simulink subsystem "PvtSubSys_VSM_TLS"  (R2020b)
settings: Solver=VariableStepAuto  StartTime=0.0  StopTime=10.0  RelTol=1e-3
undefined symbols (not defined in the file or in its folder): HWA_STATE, LCK_STATE, P_VSM_TLS_LCCancelTime
libraries: simulink x18
settings Model: Creator=GW00133806  LastModifiedBy=GW00201118

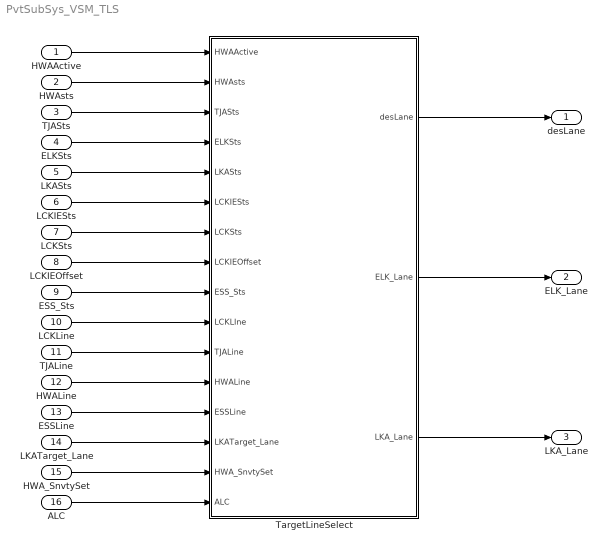
== system PvtSubSys_VSM_TLS ==
  HWAActive : Inport  Description=b|HWA激活状态
  HWAsts : Inport  Description=|  Port=2  OutDataTypeStr=Enum: HWA_STATE
      | uint8|HWA状态：0-OFF;1-Idle;2-Ready;3-CCAct（巡航）;4-Pause;5-LeftTurn;6-RightTurn;
      | 7-Error;9-SafeStop;10-SlowRetreat
  TJASts : Inport  Description=|  Port=3  OutDataTypeStr=Enum: TJA_STATE
      | uint8|TJS状态：0-Off;1-Idle;2-Ready;3-Active;6-wait;7-Error;9-SafeStop;
      | 10-SlowRetreat.
  "ELKSts " : Inport  Description=|  Port=4  OutDataTypeStr=Enum: ELKSTATE
      | uint8|ELK状态：0-ELK_OFF;1-ELK_IDLE;2-ELK_READY;3_ELK_ACTIVE_LEFT;4-ELK_ACTIVE_RIGHT;
      | 5-ELK_OnComing_LEFT;6-ELK_OnComing_RIGHT;7-ELK_OVERTAKING_LEFT;
      | 8-ELK_OVERTAKING_RIGHT;9-ELK_ERROR;10-ELK_DEFAULT;
  LKASts : Inport  Description=|  Port=5  OutDataTypeStr=Enum: STATE
      | uint8|LKA状态：0-OFF;1-IDLE;2-READY;3-ACTIVE;4-ACTIVE_LEFT;5-ACTIVE_RIGHT;
      | 6-ERROR;7-DEFAULT.
  LCKIESts : Inport  Description=|  Port=6  OutDataTypeStr=Enum: STATE
      | uint8|LCKIE状态：0-OFF;1-IDLE;2-READY;3-ACTIVE;4-ACTIVE_LEFT;5-ACTIVE_RIGHT;
      | 6-ERROR;7-DEFAULT.
  LCKSts : Inport  Description=uint8|LCK状态：0-LCK_OFF;1-LCK_Idle;2-LCK_Ready;3-LCK_Active;7-LCK_Errror.  Port=7  OutDataTypeStr=Enum: LCK_STATE
  LCKIEOffset : Inport  Description=m|LCKIE车道线C0偏移量  Port=8
  "ESS_Sts " : Inport  Description=|  Port=9
      | uint8|ESS状态：0-Off;1-IDLE;2-Ready;3-Active;4-Active_LEFT;5-Active_Right;
      | 6-Error.
  LCKLine : Inport  Port=10  OutDataTypeStr=Bus: LSM_LCK_BUS
  TJALine : Inport  Port=11  OutDataTypeStr=Bus: LSM_TJA_ICA_BUS
  HWALine : Inport  Port=12  OutDataTypeStr=Bus: LSM_HWA_BUS
  ESSLine : Inport  Port=13  OutDataTypeStr=Bus: LSM_ESS_BUS
  "LKATarget_Lane " : Inport  Port=14  OutDataTypeStr=Bus: LaneARe_SP
  HWA_SnvtySet : Inport  Description=uint8|HWA换道灵敏度  Port=15
  ALC : Inport  Description=|  Port=16
      | bus|PLAN发的总线信号："HMI提示信息驱动信号；0x1 换道完成请关闭转向灯
      | 0x2 换道取消;0x3 换道超时;0x4 换道速度过低;0x5 即将向左超车;0x6 即将向右超车
      | 0x7 车速过高不可换道"
  TargetLineSelect : Subsystem
  desLane : Outport  Description=|目标车道线信息  OutDataTypeStr=Bus: TLS_DesLane
  ELK_Lane : Outport  Description=|ELK车道线信息  Port=2  OutDataTypeStr=Bus: TLS_ELKLane
  LKA_Lane : Outport  Description=|LKA车道线信息  Port=3  OutDataTypeStr=Bus: TLS_LKALane
  wires:
  HWAActive/1 -> TargetLineSelect/1(HWAActive)
  HWAsts/1 -> TargetLineSelect/2(HWAsts)
  TargetLineSelect/3(LKA_Lane) -> LKA_Lane/1
  "ESS_Sts "/1 -> TargetLineSelect/9("ESS_Sts ")
  "LKATarget_Lane "/1 -> TargetLineSelect/14("LKATarget_Lane ")
  TJASts/1 -> TargetLineSelect/3(TJASts)
  LKASts/1 -> TargetLineSelect/5(LKASts)
  LCKLine/1 -> TargetLineSelect/10(LCKLIne)
  LCKSts/1 -> TargetLineSelect/7(LCKSts)
  LCKIESts/1 -> TargetLineSelect/6(LCKIESts)
  LCKIEOffset/1 -> TargetLineSelect/8(LCKIEOffset)
  TJALine/1 -> TargetLineSelect/11(TJALine)
  TargetLineSelect/2(ELK_Lane) -> ELK_Lane/1
  "ELKSts "/1 -> TargetLineSelect/4("ELKSts ")
  TargetLineSelect/1(desLane) -> desLane/1
  ESSLine/1 -> TargetLineSelect/13(ESSLine)
  HWALine/1 -> TargetLineSelect/12(HWALine)
  HWA_SnvtySet/1 -> TargetLineSelect/15(HWA_SnvtySet)
  ALC/1 -> TargetLineSelect/16(ALC)

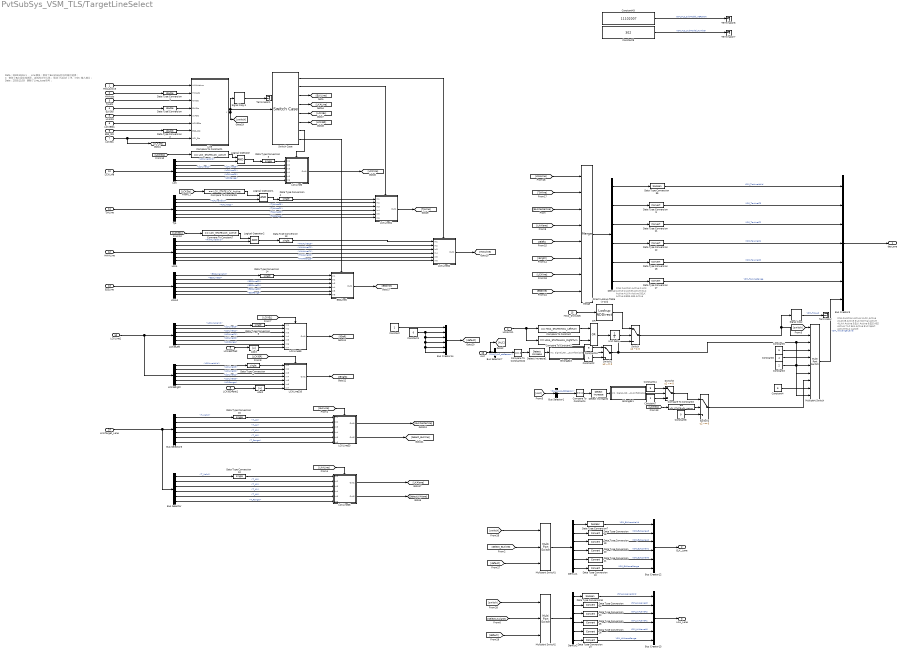
== system PvtSubSys_VSM_TLS/TargetLineSelect ==
  note: 0:No Function Active
      | 1:LCK Active
      | 2:LCKIE Active
      | 3:LC Normal Active
      | 4:LKA Active
      | 5:ELK Active
      | 6:ESS AES Active
      | 7:LC Eco Active
      | 8:LC Sport Active
      | 9:LC cancel
  note: Data：2020/10/15
      | 1、Line模块：修改了ELKstate对应的输出选择；
      | 2、修改了ELK目标线选择，边线改为中心线；
      | 取消了fusion（re、line）输入接口；
      | Data：2020/11/03
      | 删除了Line_type信号；
  note: 0:No Function Active
      | 1:LCK Active
      | 2:LCKIE Active
      | 3:LC Active
      | 4:LKA Active
      | 5:ELK Active
      | 6:ESS AES Active
  HWAActive : Inport  OutDataTypeStr=boolean
  HWAsts : Inport  Port=2
  TJASts : Inport  Port=3
  "ELKSts " : Inport  Port=4
  LKASts : Inport  Port=5
  LCKIESts : Inport  Port=6
  LCKSts : Inport  Port=7
  LCKIEOffset : Inport  Port=8  OutDataTypeStr=single
  "ESS_Sts " : Inport  Port=9  OutDataTypeStr=uint8
  LCKLIne : Inport  Port=10
  TJALine : Inport  Port=11
  HWALine : Inport  Port=12
  ESSLine : Inport  Port=13
  "LKATarget_Lane " : Inport  Port=14
  HWA_SnvtySet : Inport  Port=15
  ALC : Inport  Port=16
  Abs2 : Abs
  Abs3 : Abs
  Bus Creator12 : BusCreator  Inputs=6
  Bus Creator13 : BusCreator  Inputs=6
  Bus Creator14 : BusCreator  Inputs=6
  Bus Selector : BusSelector  OutputSignals=T_Valid,T_A3,T_A2,T_A1,T_A0,T_Range
  Bus Selector1 : BusSelector  OutputSignals=PLAN_ALC_stsReason
  Bus Selector3 : BusSelector  OutputSignals=T_Valid,T_A3,T_A2,T_A1,T_A0,T_Range
  Bus Selector7 : BusSelector  OutputSignals=PLAN_ALC_stsReason
  Bus Creator3 : BusCreator  Inputs=7
  Compare To Constant : simulink/Logic and Bit Operations/Compare To Constant  relop===  const=HWA_STATE.HWA_LeftTurn  OutDataTypeStr=boolean
  Compare To Constant{1,3,6..7} (4 alike) : simulink/Logic and Bit Operations/Compare To Constant  relop===  const=LCK_STATE.LCK_Active  OutDataTypeStr=boolean
  Compare To Constant102 : simulink/Logic and Bit Operations/Compare To Constant  relop===  const=2  OutDataTypeStr=boolean
  Compare To Constant2 : simulink/Logic and Bit Operations/Compare To Constant  relop===  const=HWA_STATE.HWA_RightTurn  OutDataTypeStr=boolean
  Compare To Constant4 : simulink/Logic and Bit Operations/Compare To Constant  relop===  const=2  OutDataTypeStr=boolean
  Constant : Constant  OutDataTypeStr=single
  Constant1 : Constant  Value=0  OutDataTypeStr=single
  Constant10 : Constant  Value=9  OutDataTypeStr=uint8
  Constant11 : Constant  Value=9  OutDataTypeStr=uint8
  Constant2 : Constant  OutDataTypeStr=uint8
  Constant3 : Constant  Value=2  OutDataTypeStr=uint8
  Constant4 : Constant  Value=6  OutDataTypeStr=uint8
  Constant43 : Constant  Value=11102007  OutDataTypeStr=uint32
  Constant5 : Constant  Value=5  OutDataTypeStr=uint8
  Constant6 : Constant  Value=4  OutDataTypeStr=uint8
  Constant7 : Constant  OutDataTypeStr=uint8
  Constant8 : Constant  Value=0  OutDataTypeStr=uint8
  Constant9 : Constant  Value=302  OutDataTypeStr=uint16
  Data Type Conversion : DataTypeConversion  OutDataTypeStr=double
  Data Type Conversion1 : DataTypeConversion  OutDataTypeStr=double
  Data Type Conversion{3..6,10,13..15} (8 alike) : DataTypeConversion  OutDataTypeStr=single
  Data Type Conversion{9,11..12,16..27} (15 alike) : DataTypeConversion
  Data Type Conversion2 : DataTypeConversion  OutDataTypeStr=double
  Data Type Conversion35 : DataTypeConversion  OutDataTypeStr=boolean
  Data Type Conversion7 : DataTypeConversion  OutDataTypeStr=boolean
  Data Type Conversion8 : DataTypeConversion  OutDataTypeStr=boolean
  Demux : Demux  Outputs=6
  Demux1 : Demux  Outputs=6
  Demux2 : Demux  Outputs=6
  Detect Increase1 : simulink/Logic and Bit Operations/Detect Increase  vinit=0.0  OutDataTypeStr=boolean
  Detect Increase2 : simulink/Logic and Bit Operations/Detect Increase  vinit=0.0  OutDataTypeStr=boolean
  Direct Lookup Table (n-D)2 : LookupNDDirect  NumberOfTableDimensions=1  Table=[3 8 7]  TableDataTypeStr=uint8
  ESSLineS : Subsystem  TreatAsAtomicUnit=on
  Enlong3s1 : Subsystem
  Enlong3s3 : Subsystem
  HWA : BusSelector  OutputSignals=HWALineValid,HWALineC3,HWALineC2,HWALineC1,HWALineC0,HWARange
  HWA2 : BusSelector  OutputSignals=ESSLineValid,ESSLineC3,ESSLineC2,ESSLineC1,ESSLineC0,ESSRange
  HWAsts1 : InportShadow  Port=2
  LCK : BusSelector  OutputSignals=LCKLineValid,LCKLineC3,LCKLineC2,LCKLineC1,LCKLineC0,LCKRange
  LCKIELeft : BusSelector  OutputSignals=LCKLineValid,LCKLineC3,LCKLineC2,LCKLineC1,LCKLineC0,LCKRange
  LCKIEOffset1 : InportShadow  Port=8  OutDataTypeStr=single
  LCKIERight : BusSelector  OutputSignals=LCKLineValid,LCKLineC3,LCKLineC2,LCKLineC1,LCKLineC0,LCKRange
  LCKLIne1 : InportShadow  Port=10
  LCKLineS : Subsystem  TreatAsAtomicUnit=on
  LCKLineS1 : Subsystem  TreatAsAtomicUnit=on
  LCKLineS10 : Subsystem  TreatAsAtomicUnit=on
  LCKLineS2 : Subsystem  TreatAsAtomicUnit=on
  LCKLineS3 : Subsystem  TreatAsAtomicUnit=on
  LCKLineS6 : Subsystem  TreatAsAtomicUnit=on
  LCKLineS9 : Subsystem  TreatAsAtomicUnit=on
  Line : MATLAB Function  TreatAsAtomicUnit=on
  Logical Operator : Logic  AllPortsSameDT=off  OutDataTypeStr=boolean
  Logical Operator1 : Logic  AllPortsSameDT=off  OutDataTypeStr=boolean
  Logical Operator2 : Logic  AllPortsSameDT=off  OutDataTypeStr=boolean
  Merge : Merge  Inputs=8
  Multiport Switch : MultiPortSwitch  Inputs=9
  Multiport Switch1 : MultiPortSwitch  DataPortOrder=Specify indices  Inputs=4  DataPortIndices={3,7}  DiagnosticForDefault=None
  Multiport Switch2 : MultiPortSwitch  DataPortOrder=Specify indices  Inputs=4  DataPortIndices={7,8}  DiagnosticForDefault=None
  OR : Logic  Operator=OR  AllPortsSameDT=off  OutDataTypeStr=boolean
  Signal Copy : SignalConversion  OverrideOpt=off
  Signal Copy1 : SignalConversion  OverrideOpt=off
  Switch{,1..3} (4 alike) : Switch  Criteria=u2 ~= 0
  Switch Case : SwitchCase  CaseConditions={1,2,3,4,5,6,7,8}  ShowDefaultCase=off
  TJA : BusSelector  OutputSignals=TJALineValid,TJALineC3,TJALineC2,TJALineC1,TJALineC0,TJARange
  Terminator{,1,6..7} (4 alike) : Terminator
  Unit Delay : UnitDelay  SampleTime=-1  HasFrameUpgradeWarning=on
  desLane : Outport
  ELK_Lane : Outport  Port=2
  LKA_Lane : Outport  Port=3
  wires:
  Constant2/1 -> Switch2/3
  Detect Increase1/1 -> Enlong3s3/1(In1)
  Constant10/1 -> Switch2/1
  Enlong3s3/1(Signal_NOH_SysInfoDisplay) -> Switch2/2
  Bus Selector7/1 -> Compare To Constant102/1  "<PLAN_ALC_stsReason>"
  ALC/1 -> Bus Selector7/1, [ALC]
  Compare To Constant102/1 -> Detect Increase1/1
  Switch3/1 -> Switch1/1
  Constant7/1 -> Switch3/3
  Detect Increase2/1 -> Enlong3s1/1(In1)
  Constant11/1 -> Switch3/1
  Enlong3s1/1(Signal_NOH_SysInfoDisplay) -> Switch3/2
  Bus Selector1/1 -> Compare To Constant4/1  "<PLAN_ALC_stsReason>"
  [ALC] -> Bus Selector1/1
  Compare To Constant4/1 -> Detect Increase2/1
  Signal Copy1/1 -> Terminator1/1
  Signal Copy/1 -> Terminator/1  "VSM_TLS_LC"
  Switch/1 -> Multiport Switch/2, Signal Copy/1
  Constant43/1 -> Terminator6/1  "VSM_TLS_SubModel_VERSION"
  Constant9/1 -> Terminator7/1  "VSM_TLS_SubModel_Number"
  HWA_SnvtySet/1 -> Direct Lookup Table (n-D)2/1
  Data Type Conversion8/1 -> Bus Creator13/1  "VSM_LKALaneValid"
  Data Type Conversion7/1 -> Bus Creator12/1  "VSM_ELKLaneValid"
  Data Type Conversion2/1 -> Line/7(ESS_Sts)
  LCKLIne1/1 -> LCKIELeft/1, LCKIERight/1
  ESSLine/1 -> HWA2/1
  HWALine/1 -> HWA/1
  TJALine/1 -> TJA/1
  [SelectLKAlane] -> Multiport Switch2/2
  LCKLineS6/2(Out2) -> [SelectLKAlane]
  Demux/1 -> Data Type Conversion35/1
  Switch Case/7 -> LCKLineS/Action
  Data Type Conversion10/1 -> LCKLineS6/1(In1)
  Bus Selector/6 -> LCKLineS6/6(In6)  "<T_Range>"
  Bus Selector/5 -> LCKLineS6/5(In5)  "<T_A0>"
  Bus Selector/4 -> LCKLineS6/4(In4)  "<T_A1>"
  Bus Selector/3 -> LCKLineS6/3(In3)  "<T_A2>"
  Bus Selector/2 -> LCKLineS6/2(In2)  "<T_A3>"
  Bus Selector/1 -> Data Type Conversion10/1  "<T_Valid>"
  ESSLineS/1(Out1) -> [ESSline]
  Data Type Conversion14/1 -> ESSLineS/1(In1)
  Switch Case/8 -> ESSLineS/Action
  HWA2/6 -> ESSLineS/6(In6)  "<ESSRange>"
  HWA2/5 -> ESSLineS/5(In5)  "<ESSLineC0>"
  HWA2/4 -> ESSLineS/4(In4)  "<ESSLineC1>"
  HWA2/3 -> ESSLineS/3(In3)  "<ESSLineC2>"
  HWA2/2 -> ESSLineS/2(In2)  "<ESSLineC3>"
  HWA2/1 -> Data Type Conversion14/1  "<ESSLineValid>"
  "ESS_Sts "/1 -> Data Type Conversion2/1
  LCKLineS3/2(Out2) -> [Select_ELKline]
  [ELKCenterline] -> Merge/3
  [TJAline] -> Merge/2
  [HWAline] -> Merge/1
  Merge/1 -> Demux/1
  LCKLineS6/1(Out1) -> [LKAlane]
  LCKLineS3/1(Out1) -> [ELKCenterline]
  LCKLineS10/1(Out1) -> [IEright]
  LCKLineS9/1(Out1) -> [IEleft]
  LCKLineS2/1(Out1) -> [HWAline]
  LCKLineS1/1(Out1) -> [TJAline]
  LCKLineS/1(Out1) -> [LCKline]
  [default] -> Multiport Switch2/3
  [switch] -> Multiport Switch2/1
  [default] -> Multiport Switch1/3
  Bus Creator14/1 -> [default]
  Constant1/1 -> Bus Creator14/2, Bus Creator14/4, Bus Creator14/6, Bus Creator14/5, Bus Creator14/3
  Constant/1 -> Bus Creator14/1
  [switch] -> Multiport Switch1/1
  Line/1(y) -> [switch], Switch Case/1, Signal Copy1/1
  Data Type Conversion3/1 -> LCKLineS/1(In1)
  Logical Operator/1 -> Data Type Conversion3/1
  Bus Creator12/1 -> ELK_Lane/1
  LCK/1 -> Logical Operator/2  "<LCKLineValid>"
  Bus Creator13/1 -> LKA_Lane/1
  Demux2/6 -> Data Type Conversion27/1
  Demux2/5 -> Data Type Conversion26/1
  Demux2/4 -> Data Type Conversion25/1
  Demux2/3 -> Data Type Conversion24/1
  Demux2/2 -> Data Type Conversion23/1
  Demux2/1 -> Data Type Conversion8/1
  Multiport Switch2/1 -> Demux2/1
  Demux1/6 -> Data Type Conversion22/1
  Demux1/5 -> Data Type Conversion21/1
  Demux1/4 -> Data Type Conversion20/1
  Demux1/3 -> Data Type Conversion19/1
  Demux1/2 -> Data Type Conversion18/1
  Demux1/1 -> Data Type Conversion7/1
  Multiport Switch1/1 -> Demux1/1
  [Select_ELKline] -> Multiport Switch1/2
  Abs3/1 -> LCKLineS9/7(In7)
  Abs2/1 -> LCKLineS10/7(In7)
  Data Type Conversion1/1 -> Line/2(HWAsts)
  HWAsts/1 -> Data Type Conversion1/1
  LCKIEOffset/1 -> Abs3/1
  Data Type Conversion35/1 -> Bus Creator3/1  "VSM_TarLineValid"
  Data Type Conversion13/1 -> LCKLineS2/1(In1)
  Data Type Conversion6/1 -> LCKLineS10/1(In1)
  Data Type Conversion5/1 -> LCKLineS9/1(In1)
  Data Type Conversion4/1 -> LCKLineS1/1(In1)
  Compare To Constant1/1 -> Logical Operator/1
  [LCKIER] -> LCKLineS10/Action
  [LCKIEL] -> LCKLineS9/Action
  [LKALine] -> LCKLineS6/Action
  [ELKLine] -> LCKLineS3/Action
  Switch Case/3 -> [ELKLine]
  Data Type Conversion/1 -> Line/4(ELKSts)
  LCKIESts/1 -> Line/6(LCKIESts)
  LKASts/1 -> Line/5(LKASts)
  "ELKSts "/1 -> Data Type Conversion/1
  LCKIEOffset1/1 -> Abs2/1
  LCKIERight/6 -> LCKLineS10/6(In6)  "<LCKRange>"
  LCKIERight/4 -> LCKLineS10/4(In4)  "<LCKLineC1>"
  LCKIERight/3 -> LCKLineS10/3(In3)  "<LCKLineC2>"
  LCKIERight/1 -> Data Type Conversion6/1  "<LCKLineValid>"
  LCKIERight/5 -> LCKLineS10/5(In5)  "<LCKLineC0>"
  LCKIERight/2 -> LCKLineS10/2(In2)  "<LCKLineC3>"
  LCKIELeft/6 -> LCKLineS9/6(In6)  "<LCKRange>"
  LCKIELeft/1 -> Data Type Conversion5/1  "<LCKLineValid>"
  LCKIELeft/3 -> LCKLineS9/3(In3)  "<LCKLineC2>"
  LCKIELeft/5 -> LCKLineS9/5(In5)  "<LCKLineC0>"
  LCKIELeft/2 -> LCKLineS9/2(In2)  "<LCKLineC3>"
  LCKIELeft/4 -> LCKLineS9/4(In4)  "<LCKLineC1>"
  LCKLIne/1 -> LCK/1
  LCK/6 -> LCKLineS/6(In6)  "<LCKRange>"
  LCK/2 -> LCKLineS/2(In2)  "<LCKLineC3>"
  LCK/4 -> LCKLineS/4(In4)  "<LCKLineC1>"
  LCK/5 -> LCKLineS/5(In5)  "<LCKLineC0>"
  LCK/3 -> LCKLineS/3(In3)  "<LCKLineC2>"
  TJA/5 -> LCKLineS1/5(In5)  "<TJALineC0>"
  TJA/4 -> LCKLineS1/4(In4)  "<TJALineC1>"
  TJA/2 -> LCKLineS1/2(In2)  "<TJALineC3>"
  TJA/1 -> Logical Operator1/2  "<TJALineValid>"
  TJA/6 -> LCKLineS1/6(In6)  "<TJARange>"
  TJA/3 -> LCKLineS1/3(In3)  "<TJALineC2>"
  HWA/1 -> Logical Operator2/2  "<HWALineValid>"
  HWA/5 -> LCKLineS2/5(In5)  "<HWALineC0>"
  HWA/3 -> LCKLineS2/3(In3)  "<HWALineC2>"
  HWA/2 -> LCKLineS2/2(In2)  "<HWALineC3>"
  HWA/6 -> LCKLineS2/6(In6)  "<HWARange>"
  Demux/3 -> Data Type Conversion11/1
  HWA/4 -> LCKLineS2/4(In4)  "<HWALineC1>"
  Demux/2 -> Data Type Conversion9/1
  Switch Case/1 -> LCKLineS2/Action
  Switch Case/2 -> LCKLineS1/Action
  Demux/4 -> Data Type Conversion12/1
  Bus Creator3/1 -> desLane/1
  HWAActive/1 -> Line/1(HWAActive)
  TJASts/1 -> Line/3(TJASts)
  Demux/5 -> Data Type Conversion16/1
  Demux/6 -> Data Type Conversion17/1
  Compare To Constant6/1 -> Logical Operator1/1
  Logical Operator1/1 -> Data Type Conversion4/1
  Compare To Constant7/1 -> Logical Operator2/1
  Logical Operator2/1 -> Data Type Conversion13/1
  "LKATarget_Lane "/1 -> Bus Selector3/1, Bus Selector/1
  Bus Selector3/1 -> Data Type Conversion15/1  "<T_Valid>"
  Bus Selector3/2 -> LCKLineS3/2(In2)  "<T_A3>"
  Bus Selector3/3 -> LCKLineS3/3(In3)  "<T_A2>"
  Bus Selector3/4 -> LCKLineS3/4(In4)  "<T_A1>"
  Bus Selector3/5 -> LCKLineS3/5(In5)  "<T_A0>"
  Bus Selector3/6 -> LCKLineS3/6(In6)  "<T_Range>"
  Switch Case/4 -> [LKALine]
  Switch Case/5 -> [LCKIEL]
  Switch Case/6 -> [LCKIER]
  [LKAlane] -> Merge/4
  [IEleft] -> Merge/5
  [IEright] -> Merge/6
  [LCKline] -> Merge/7
  [ESSline] -> Merge/8
  Data Type Conversion15/1 -> LCKLineS3/1(In1)
  Multiport Switch/1 -> Bus Creator3/7  "VSM_TarDangerLevel"
  Switch2/1 -> Multiport Switch/3, Multiport Switch/10, Switch/3
  Constant3/1 -> Multiport Switch/7, Multiport Switch/6
  Constant4/1 -> Multiport Switch/9
  Constant5/1 -> Multiport Switch/4
  Constant6/1 -> Multiport Switch/5
  LCKSts/1 -> [LCKSts], Line/8(LCK_Sts)
  [LCKSts] -> Compare To Constant1/1
  [LCKSts] -> Compare To Constant6/1
  [LCKSts] -> Compare To Constant7/1
  Data Type Conversion9/1 -> Bus Creator3/2  "VSM_TarLineC3"
  Data Type Conversion11/1 -> Bus Creator3/3  "VSM_TarLineC2"
  Data Type Conversion12/1 -> Bus Creator3/4  "VSM_TarLineC1"
  Data Type Conversion16/1 -> Bus Creator3/5  "VSM_TarLineC0"
  Data Type Conversion17/1 -> Bus Creator3/6  "VSM_TarLineRange"
  Data Type Conversion18/1 -> Bus Creator12/2  "VSM_ELKLaneA3"
  Data Type Conversion19/1 -> Bus Creator12/3  "VSM_ELKLaneA2"
  Data Type Conversion20/1 -> Bus Creator12/4  "VSM_ELKLaneA1"
  Data Type Conversion21/1 -> Bus Creator12/5  "VSM_ELKLaneA0"
  Data Type Conversion22/1 -> Bus Creator12/6  "VSM_ELKLaneRange"
  Data Type Conversion23/1 -> Bus Creator13/2  "VSM_LKALaneA3"
  Data Type Conversion24/1 -> Bus Creator13/3  "VSM_LKALaneA2"
  Data Type Conversion25/1 -> Bus Creator13/4  "VSM_LKALaneA1"
  Data Type Conversion26/1 -> Bus Creator13/5  "VSM_LKALaneA0"
  Data Type Conversion27/1 -> Bus Creator13/6  "VSM_LKALaneRange"
  [switch] -> Multiport Switch/1
  HWAsts1/1 -> Compare To Constant2/1, Compare To Constant/1
  Compare To Constant/1 -> OR/1
  Compare To Constant2/1 -> OR/2
  OR/1 -> Unit Delay/1
  Direct Lookup Table (n-D)2/1 -> Switch/1
  [LCKSts] -> Compare To Constant3/1
  Compare To Constant3/1 -> Switch1/2
  Switch1/1 -> Multiport Switch/8
  Constant8/1 -> Switch1/3
  Unit Delay/1 -> Switch/2

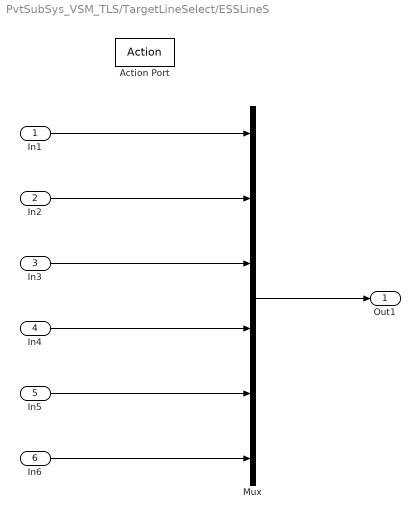
== system PvtSubSys_VSM_TLS/TargetLineSelect/ESSLineS ==
  In1 : Inport
  In2 : Inport  Port=2
  In3 : Inport  Port=3
  In4 : Inport  Port=4
  In5 : Inport  Port=5
  In6 : Inport  Port=6
  Action Port : ActionPort
  Mux : Mux  Inputs=6
  Out1 : Outport
  wires:
  In5/1 -> Mux/5
  In4/1 -> Mux/4
  In6/1 -> Mux/6
  In3/1 -> Mux/3
  In2/1 -> Mux/2
  In1/1 -> Mux/1
  Mux/1 -> Out1/1

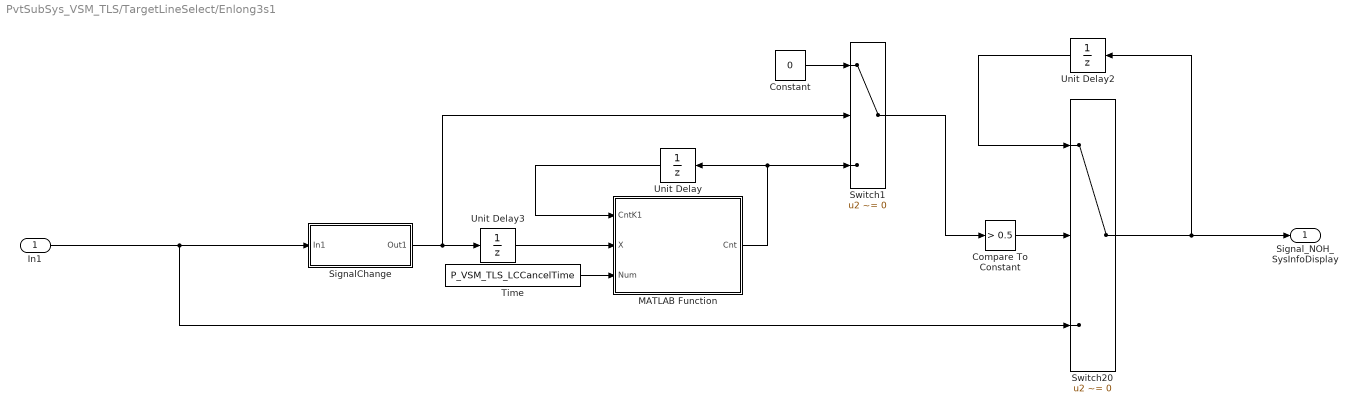
== system PvtSubSys_VSM_TLS/TargetLineSelect/Enlong3s1 ==
  In1 : Inport
  Compare To Constant : simulink/Logic and Bit Operations/Compare To Constant  relop=>  const=0.5  OutDataTypeStr=boolean
  Constant : Constant  Value=0  OutDataTypeStr=uint16
  MATLAB Function : MATLAB Function  TreatAsAtomicUnit=on
  SignalChange : Subsystem
  Switch1 : Switch  Criteria=u2 ~= 0
  Switch20 : Switch  Criteria=u2 ~= 0
  Time : Constant  Description=250  Value=P_VSM_TLS_LCCancelTime  OutDataTypeStr=uint16
      settings: AttributesFormatString=%<Description>
  Unit Delay : UnitDelay  SampleTime=-1  HasFrameUpgradeWarning=on
  Unit Delay2 : UnitDelay  SampleTime=-1  HasFrameUpgradeWarning=on
  Unit Delay3 : UnitDelay  SampleTime=-1  HasFrameUpgradeWarning=on
  Signal_NOH_SysInfoDisplay : Outport
  wires:
  In1/1 -> Switch20/3, SignalChange/1(In1)
  SignalChange/1(Out1) -> Switch1/2, Unit Delay3/1
  Unit Delay/1 -> MATLAB Function/1(CntK1)
  Constant/1 -> Switch1/1
  MATLAB Function/1(Cnt) -> Switch1/3, Unit Delay/1
  Switch1/1 -> Compare To Constant/1
  Compare To Constant/1 -> Switch20/2
  Unit Delay3/1 -> MATLAB Function/2(X)
  Unit Delay2/1 -> Switch20/1
  Switch20/1 -> Unit Delay2/1, Signal_NOH_SysInfoDisplay/1
  Time/1 -> MATLAB Function/3(Num)

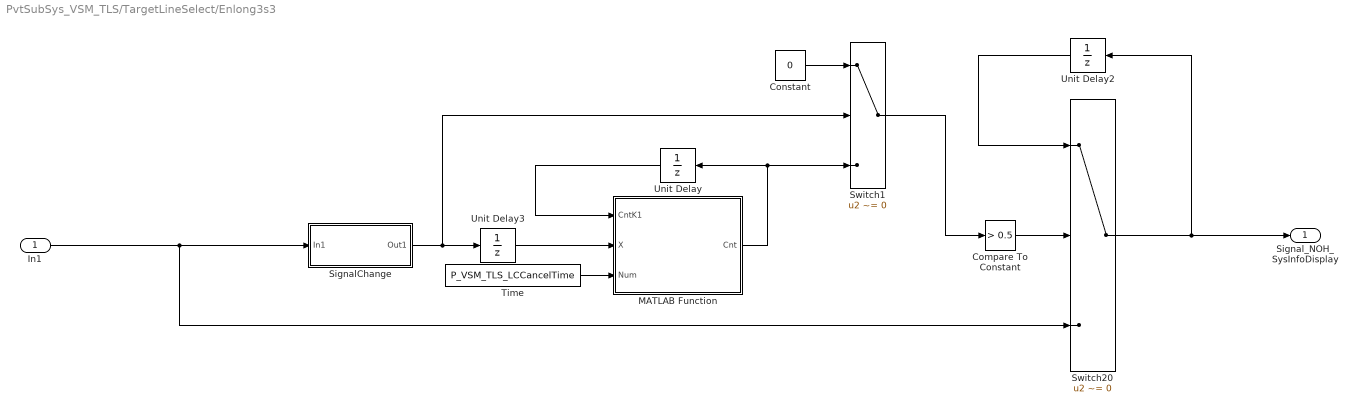
== system PvtSubSys_VSM_TLS/TargetLineSelect/Enlong3s3 ==
  In1 : Inport
  Compare To Constant : simulink/Logic and Bit Operations/Compare To Constant  relop=>  const=0.5  OutDataTypeStr=boolean
  Constant : Constant  Value=0  OutDataTypeStr=uint16
  MATLAB Function : MATLAB Function  TreatAsAtomicUnit=on
  SignalChange : Subsystem
  Switch1 : Switch  Criteria=u2 ~= 0
  Switch20 : Switch  Criteria=u2 ~= 0
  Time : Constant  Description=250  Value=P_VSM_TLS_LCCancelTime  OutDataTypeStr=uint16
      settings: AttributesFormatString=%<Description>
  Unit Delay : UnitDelay  SampleTime=-1  HasFrameUpgradeWarning=on
  Unit Delay2 : UnitDelay  SampleTime=-1  HasFrameUpgradeWarning=on
  Unit Delay3 : UnitDelay  SampleTime=-1  HasFrameUpgradeWarning=on
  Signal_NOH_SysInfoDisplay : Outport
  wires:
  In1/1 -> Switch20/3, SignalChange/1(In1)
  SignalChange/1(Out1) -> Switch1/2, Unit Delay3/1
  Unit Delay/1 -> MATLAB Function/1(CntK1)
  Constant/1 -> Switch1/1
  MATLAB Function/1(Cnt) -> Switch1/3, Unit Delay/1
  Switch1/1 -> Compare To Constant/1
  Compare To Constant/1 -> Switch20/2
  Unit Delay3/1 -> MATLAB Function/2(X)
  Unit Delay2/1 -> Switch20/1
  Switch20/1 -> Unit Delay2/1, Signal_NOH_SysInfoDisplay/1
  Time/1 -> MATLAB Function/3(Num)

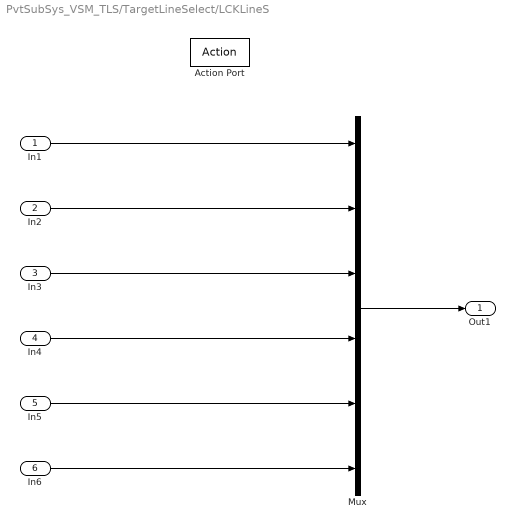
== system PvtSubSys_VSM_TLS/TargetLineSelect/LCKLineS ==
  In1 : Inport
  In2 : Inport  Port=2
  In3 : Inport  Port=3
  In4 : Inport  Port=4
  In5 : Inport  Port=5
  In6 : Inport  Port=6
  Action Port : ActionPort
  Mux : Mux  Inputs=6
  Out1 : Outport
  wires:
  In6/1 -> Mux/6
  In5/1 -> Mux/5
  In4/1 -> Mux/4
  In3/1 -> Mux/3
  Mux/1 -> Out1/1
  In2/1 -> Mux/2
  In1/1 -> Mux/1

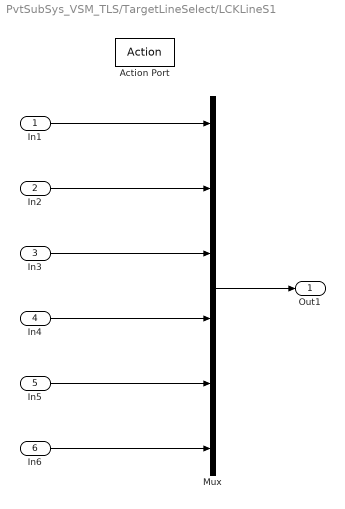
== system PvtSubSys_VSM_TLS/TargetLineSelect/LCKLineS1 ==
  In1 : Inport
  In2 : Inport  Port=2
  In3 : Inport  Port=3
  In4 : Inport  Port=4
  In5 : Inport  Port=5
  In6 : Inport  Port=6
  Action Port : ActionPort
  Mux : Mux  Inputs=6
  Out1 : Outport
  wires:
  In6/1 -> Mux/6
  In1/1 -> Mux/1
  In5/1 -> Mux/5
  In2/1 -> Mux/2
  In3/1 -> Mux/3
  In4/1 -> Mux/4
  Mux/1 -> Out1/1

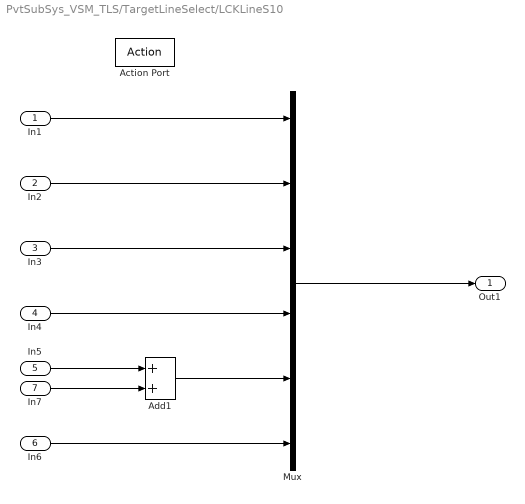
== system PvtSubSys_VSM_TLS/TargetLineSelect/LCKLineS10 ==
  In1 : Inport
  In2 : Inport  Port=2
  In3 : Inport  Port=3
  In4 : Inport  Port=4
  In5 : Inport  Port=5
  In6 : Inport  Port=6
  In7 : Inport  Port=7
  Action Port : ActionPort
  Add1 : Sum
  Mux : Mux  Inputs=6
  Out1 : Outport
  wires:
  Mux/1 -> Out1/1
  In6/1 -> Mux/6
  In1/1 -> Mux/1
  In4/1 -> Mux/4
  In2/1 -> Mux/2
  In3/1 -> Mux/3
  Add1/1 -> Mux/5
  In5/1 -> Add1/1
  In7/1 -> Add1/2

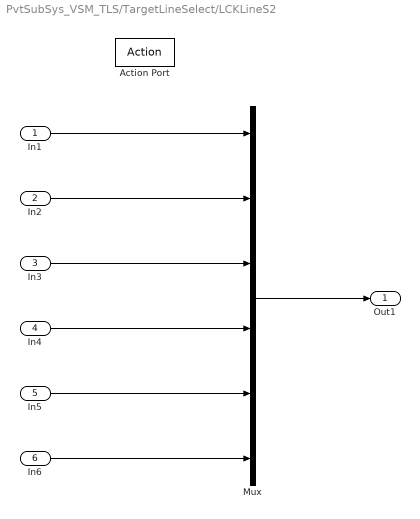
== system PvtSubSys_VSM_TLS/TargetLineSelect/LCKLineS2 ==
  In1 : Inport
  In2 : Inport  Port=2
  In3 : Inport  Port=3
  In4 : Inport  Port=4
  In5 : Inport  Port=5
  In6 : Inport  Port=6
  Action Port : ActionPort
  Mux : Mux  Inputs=6
  Out1 : Outport
  wires:
  Mux/1 -> Out1/1
  In1/1 -> Mux/1
  In2/1 -> Mux/2
  In3/1 -> Mux/3
  In6/1 -> Mux/6
  In4/1 -> Mux/4
  In5/1 -> Mux/5

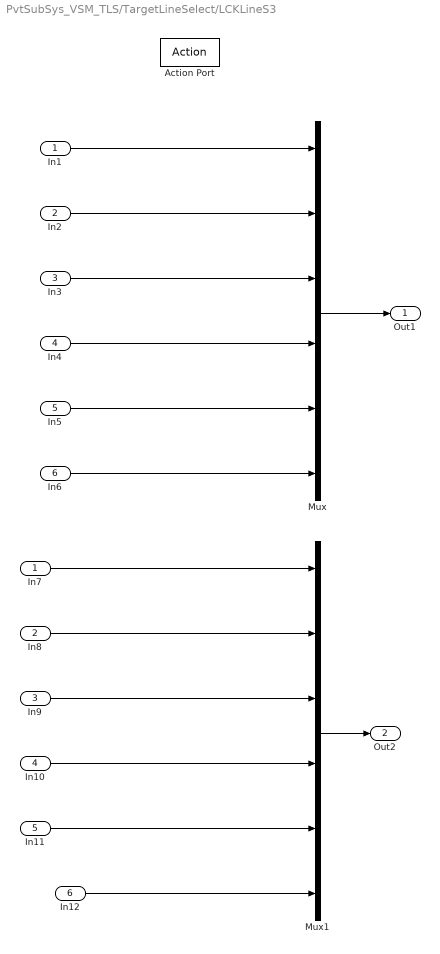
== system PvtSubSys_VSM_TLS/TargetLineSelect/LCKLineS3 ==
  In1 : Inport
  In2 : Inport  Port=2
  In3 : Inport  Port=3
  In4 : Inport  Port=4
  In5 : Inport  Port=5
  In6 : Inport  Port=6
  Action Port : ActionPort
  In10 : InportShadow  Port=4
  In11 : InportShadow  Port=5
  In12 : InportShadow  Port=6
  In7 : InportShadow
  In8 : InportShadow  Port=2
  In9 : InportShadow  Port=3
  Mux : Mux  Inputs=6
  Mux1 : Mux  Inputs=6
  Out1 : Outport
  Out2 : Outport  Port=2
  wires:
  In5/1 -> Mux/5
  In1/1 -> Mux/1
  In2/1 -> Mux/2
  In3/1 -> Mux/3
  In4/1 -> Mux/4
  In6/1 -> Mux/6
  Mux/1 -> Out1/1
  Mux1/1 -> Out2/1
  In7/1 -> Mux1/1
  In8/1 -> Mux1/2
  In9/1 -> Mux1/3
  In10/1 -> Mux1/4
  In11/1 -> Mux1/5
  In12/1 -> Mux1/6

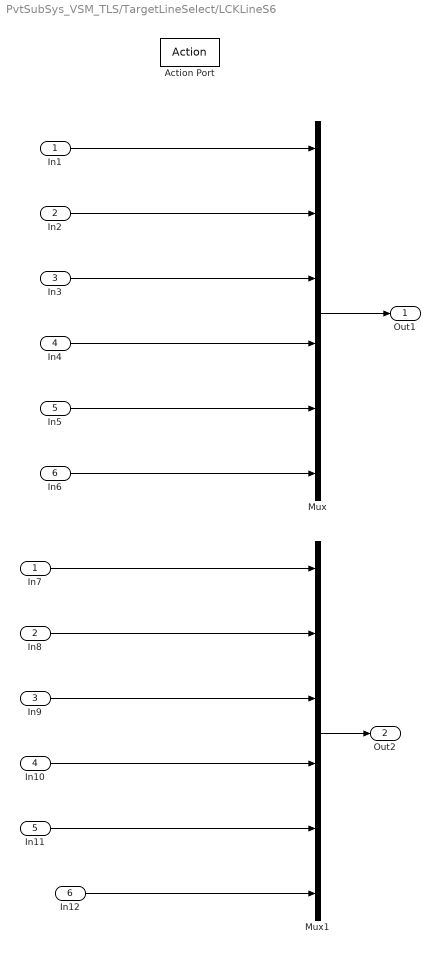
== system PvtSubSys_VSM_TLS/TargetLineSelect/LCKLineS6 ==
  In1 : Inport
  In2 : Inport  Port=2
  In3 : Inport  Port=3
  In4 : Inport  Port=4
  In5 : Inport  Port=5
  In6 : Inport  Port=6
  Action Port : ActionPort
  In10 : InportShadow  Port=4
  In11 : InportShadow  Port=5
  In12 : InportShadow  Port=6
  In7 : InportShadow
  In8 : InportShadow  Port=2
  In9 : InportShadow  Port=3
  Mux : Mux  Inputs=6
  Mux1 : Mux  Inputs=6
  Out1 : Outport
  Out2 : Outport  Port=2
  wires:
  In12/1 -> Mux1/6
  In11/1 -> Mux1/5
  In10/1 -> Mux1/4
  In9/1 -> Mux1/3
  In8/1 -> Mux1/2
  In7/1 -> Mux1/1
  Mux1/1 -> Out2/1
  Mux/1 -> Out1/1
  In6/1 -> Mux/6
  In4/1 -> Mux/4
  In3/1 -> Mux/3
  In2/1 -> Mux/2
  In1/1 -> Mux/1
  In5/1 -> Mux/5

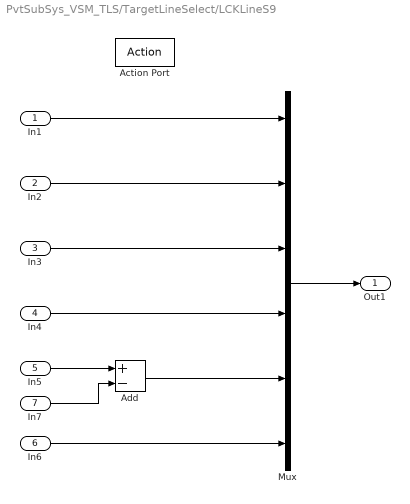
== system PvtSubSys_VSM_TLS/TargetLineSelect/LCKLineS9 ==
  In1 : Inport
  In2 : Inport  Port=2
  In3 : Inport  Port=3
  In4 : Inport  Port=4
  In5 : Inport  Port=5
  In6 : Inport  Port=6
  In7 : Inport  Port=7
  Action Port : ActionPort
  Add : Sum  Inputs=+-
  Mux : Mux  Inputs=6
  Out1 : Outport
  wires:
  Mux/1 -> Out1/1
  In6/1 -> Mux/6
  In1/1 -> Mux/1
  In4/1 -> Mux/4
  In2/1 -> Mux/2
  In3/1 -> Mux/3
  Add/1 -> Mux/5
  In7/1 -> Add/2
  In5/1 -> Add/1

== system PvtSubSys_VSM_TLS/TargetLineSelect/Enlong3s1/SignalChange ==
  In1 : Inport
  Compare To Constant1 : simulink/Logic and Bit Operations/Compare To Constant  relop=~=  const=0  OutDataTypeStr=boolean
  Detect Decrease : simulink/Logic and Bit Operations/Detect Decrease  vinit=0.0  OutDataTypeStr=boolean
  Detect Increase3 : simulink/Logic and Bit Operations/Detect Increase  vinit=0.0  OutDataTypeStr=boolean
  Logical Operator : Logic  Operator=OR  AllPortsSameDT=off  OutDataTypeStr=boolean
  Logical Operator1 : Logic  AllPortsSameDT=off  OutDataTypeStr=boolean
  Out1 : Outport
  wires:
  In1/1 -> Detect Increase3/1, Detect Decrease/1, Compare To Constant1/1
  Detect Increase3/1 -> Logical Operator/2
  Compare To Constant1/1 -> Logical Operator1/1
  Logical Operator1/1 -> Out1/1
  Logical Operator/1 -> Logical Operator1/2
  Detect Decrease/1 -> Logical Operator/1

== system PvtSubSys_VSM_TLS/TargetLineSelect/Enlong3s3/SignalChange ==
  In1 : Inport
  Compare To Constant1 : simulink/Logic and Bit Operations/Compare To Constant  relop=~=  const=0  OutDataTypeStr=boolean
  Detect Decrease : simulink/Logic and Bit Operations/Detect Decrease  vinit=0.0  OutDataTypeStr=boolean
  Detect Increase3 : simulink/Logic and Bit Operations/Detect Increase  vinit=0.0  OutDataTypeStr=boolean
  Logical Operator : Logic  Operator=OR  AllPortsSameDT=off  OutDataTypeStr=boolean
  Logical Operator1 : Logic  AllPortsSameDT=off  OutDataTypeStr=boolean
  Out1 : Outport
  wires:
  In1/1 -> Detect Increase3/1, Detect Decrease/1, Compare To Constant1/1
  Detect Increase3/1 -> Logical Operator/2
  Compare To Constant1/1 -> Logical Operator1/1
  Logical Operator1/1 -> Out1/1
  Logical Operator/1 -> Logical Operator1/2
  Detect Decrease/1 -> Logical Operator/1

== matlab function PvtSubSys_VSM_TLS/TargetLineSelect/Enlong3s3/MATLAB Function ==
  data: CntK1 input uint16; Cnt output uint16; X input; Num input
function Cnt= TextCount(CntK1,X,Num)

if X==true
    Cnt = Num;
else
     Cnt = max(CntK1-uint16(1),uint16(0));
end

== matlab function PvtSubSys_VSM_TLS/TargetLineSelect/Line ==
  data: HWAActive input; HWAsts input; y output; TJASts input; ELKSts input; LKASts input; LCKIESts input; ESS_Sts input; LCK_Sts input
function y = LineSelect(HWAActive,HWAsts, TJASts,ELKSts,LKASts,LCKIESts,ESS_Sts,LCK_Sts)
y=  7;
if HWAActive
    if LCK_Sts==LCK_STATE.LCK_Active
        y = 1;
    end
    if LCKIESts ==STATE.ACTIVE_LEFT && HWAsts~=5 && HWAsts~=6
        y= 5;
    elseif LCKIESts==STATE.ACTIVE_RIGHT && HWAsts~=5 && HWAsts~=6
        y= 6;
    end
elseif TJASts==3 || TJASts==9 || TJASts==10
    if LCK_Sts==LCK_STATE.LCK_Active
        y = 2;
    end
    if LCKIESts ==STATE.ACTIVE_LEFT && HWAsts~=5 && HWAsts~=6
        y= 5;
    elseif LCKIESts==STATE.ACTIVE_RIGHT && HWAsts~=5 && HWAsts~=6
        y= 6;
    end
elseif ELKSts==5 || ELKSts==7  %line    3:left; 4:right
    y = 3;
elseif  ELKSts==6 || ELKSts==8
    y = 3;
elseif ELKSts==3  % re                  5: left; 6: right
    y = 3;
elseif  ELKSts==4 
    y = 3;
elseif LKASts==STATE.ACTIVE_LEFT ||  LKASts==STATE.ACTIVE_RIGHT
    y =  4;
elseif ESS_Sts == 4 || ESS_Sts == 5
    y = 8;
elseif LCK_Sts==LCK_STATE.LCK_Active
    if LCKIESts ==STATE.ACTIVE_LEFT && HWAsts~=5 && HWAsts~=6
        y= 5;
    elseif LCKIESts==STATE.ACTIVE_RIGHT && HWAsts~=5 && HWAsts~=6
        y= 6;
    end    
end
end

== matlab function PvtSubSys_VSM_TLS/TargetLineSelect/Enlong3s1/MATLAB Function ==
  data: CntK1 input uint16; Cnt output uint16; X input; Num input
function Cnt= TextCount(CntK1,X,Num)

if X==true
    Cnt = Num;
else
     Cnt = max(CntK1-uint16(1),uint16(0));
end
